simulink model "motor_controller"  (R2023b)
settings: Solver=FixedStepAuto  StartTime=0.0  StopTime=10.0  RelTol=1e-3  EnableMultiTasking=on
model workspace (MAT data in the model file):
  FOC_Ts = Simulink.Parameter
  FOC_Ts.Value = 3.65714285714e-05
  FOC_Ts.DataType = 'auto'
  FOC_Ts.Complexity = 'real'
  FOC_Ts.Dimensions = [1 1]
  Outer_Ts = Simulink.Parameter
  Outer_Ts.Value = 0.001
  Outer_Ts.DataType = 'auto'
  Outer_Ts.Complexity = 'real'
  Outer_Ts.Dimensions = [1 1]
settings Model: DataDictionary=newBoard.sldd  Creator=mfussi  LastModifiedBy=mfussi
settings SolverCC: AutoInsertRateTranBlk=on  InsertRTBMode=Never (minimum delay)
settings GRTTargetCC: CodeInterfacePackaging=Reusable function  GenerateAllocFcn=on

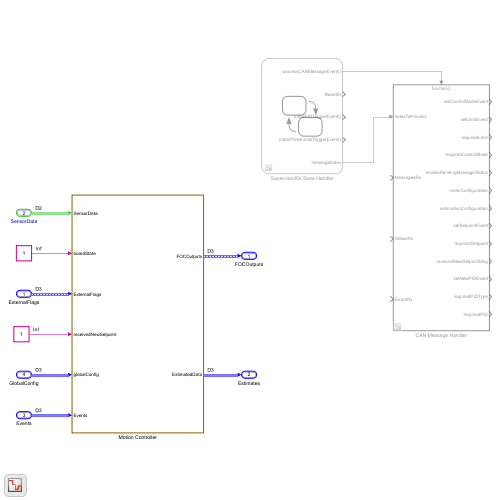
[thumbnail: Simulink's stored preview of the top-level diagram]
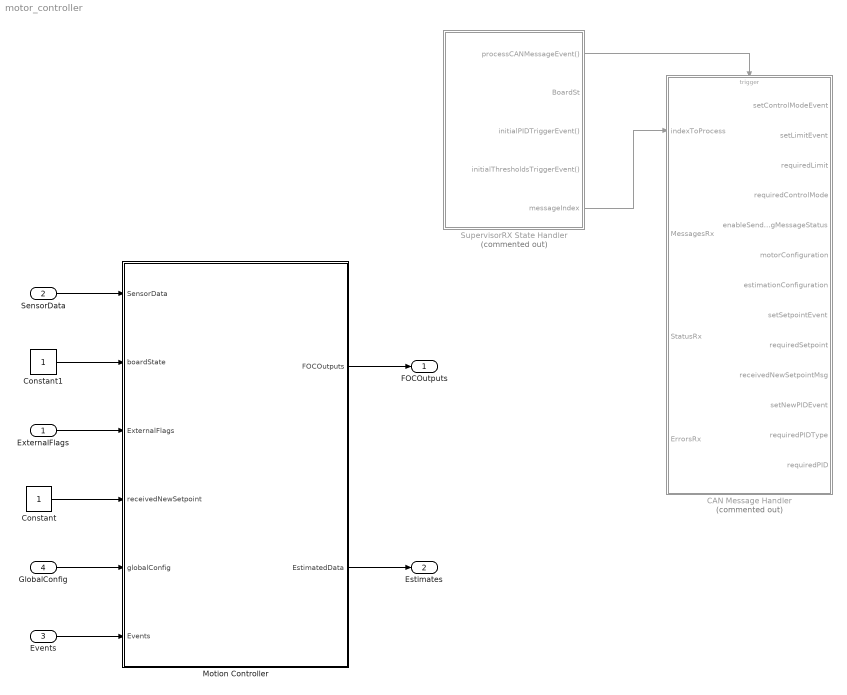
== system motor_controller ==
  ExternalFlags : Inport  OutDataTypeStr=Bus: ExternalFlags  BusOutputAsStruct=on
  SensorData : Inport  Port=2  OutDataTypeStr=Bus: SensorsData  SampleTime=FOC_Ts
  Events : Inport  Port=3  OutDataTypeStr=Bus: SupervisorReceivedEvents
  GlobalConfig : Inport  Port=4  OutDataTypeStr=Bus: GlobalConfiguration
  CAN Message Handler : Subsystem  Commented=on
  Constant : Constant  OutDataTypeStr=Inherit: Inherit via back propagation
  Constant1 : Constant
  Motion Controller : Subsystem
  SupervisorRX State Handler : Stateflow chart  Commented=on  TreatAsAtomicUnit=on
      settings: PortSchema="{\"entries\":[{\"content\":{\"sides\":[{\"content\":{},\"type\":\"ConnectorPlacement.EquallySpacedRectSide\",\"uuid\":\"4bcaed5d-410c-4a48-823b-3b1723005233\"},{\"content\":{\"connectorIds\":[\"Out3\",\"Out2\",\"Out5\",\"Out4\",\"Out1\"],\"side\":\"RIGHT\"},\"type\":\"ConnectorPlacement.EquallySpacedRectSide\",\"uuid\":\"86b3f59c-d426-4588-a6be-1a017d3ab845\"},{\"content\":{\"side\":\"TOP\"},\"type\":\"ConnectorPlacement.EquallySpacedRectSide\",\"uuid\":\"0cb05583-8f5e-45b3-ad36-5650b13dab11\"}]},\"type\":\"ConnectorPlacement.EquallySpacedConnector\",\"uuid\":\"18dc427b-0f18-405e-8b12-e70db528f537\"}],\"packageUris\":[\"http://schema.mathworks.com/mf0/Connector/R2020b\"],\"version\":\"1.0\"}"
  FOCOutputs : Outport  OutDataTypeStr=Bus: FOCOutputs
  Estimates : Outport  Port=2  OutDataTypeStr=Bus: EstimatedData
  wires:
  SupervisorRX State Handler/3(processCANMessageEvent()) -> CAN Message Handler/Trigger
  SensorData/1 -> Motion Controller/1(SensorData)
  ExternalFlags/1 -> Motion Controller/3(ExternalFlags)
  Motion Controller/1(FOCOutputs) -> FOCOutputs/1
  Motion Controller/2(EstimatedData) -> Estimates/1
  Events/1 -> Motion Controller/6(Events)
  SupervisorRX State Handler/1(messageIndex) -> CAN Message Handler/1(indexToProcess)
  GlobalConfig/1 -> Motion Controller/5(globalConfig)
  Constant/1 -> Motion Controller/4(receivedNewSetpoint)
  Constant1/1 -> Motion Controller/2(boardState)

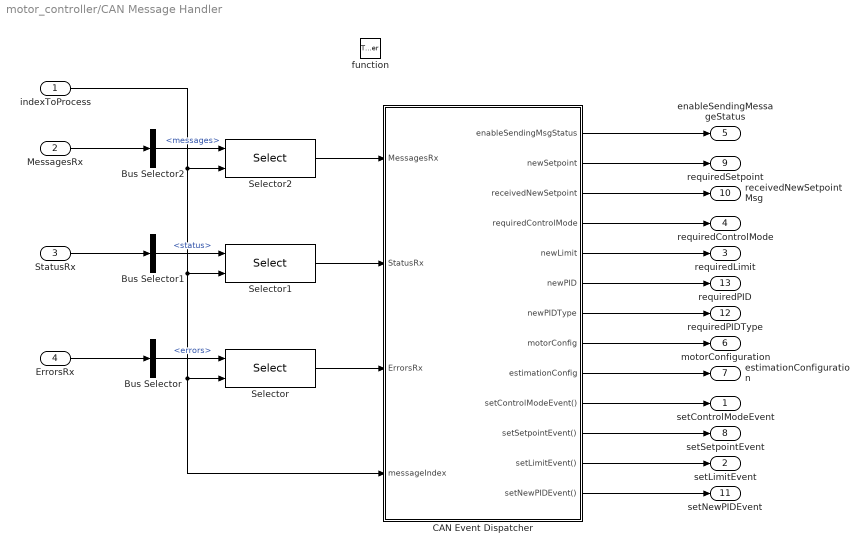
== system motor_controller/CAN Message Handler ==
  indexToProcess : Inport
  MessagesRx : Inport  Port=2  OutDataTypeStr=Bus: BUS_MESSAGES_RX_MULTIPLE
  StatusRx : Inport  Port=3  OutDataTypeStr=Bus: BUS_STATUS_RX_MULTIPLE
  ErrorsRx : Inport  Port=4  OutDataTypeStr=Bus: BUS_CAN_RX_ERRORS_MULTIPLE
  function : TriggerPort  TriggerType=function-call  VariantControl=(inherit)
  Bus Selector : BusSelector  OutputSignals=errors
  Bus Selector1 : BusSelector  OutputSignals=status
  Bus Selector2 : BusSelector  OutputSignals=messages
  CAN Event Dispatcher : Stateflow chart  TreatAsAtomicUnit=on
      settings: PortSchema="{\"entries\":[{\"content\":{\"sides\":[{\"content\":{\"connectorIds\":[\"In3\",\"In2\",\"In1\",\"In4\"]},\"type\":\"ConnectorPlacement.EquallySpacedRectSide\",\"uuid\":\"262d8322-eee9-4d2f-8394-9ad0f57315f2\"},{\"content\":{\"connectorIds\":[\"Out4\",\"Out2\",\"Out5\",\"Out1\",\"Out3\",\"Out6\",\"Out7\",\"Out8\",\"Out9\",\"Out10\",\"Out11\",\"Out12\",\"Out13\"],\"side\":\"RIGHT\"},\"type\":\"ConnectorPlacement.EquallySpacedRectSide\",\"uuid\":\"ca9d82ac-748f-4018-bf9f-4633821aba3f\"},{\"content\":{\"connectorIds\":[],\"side\":\"TOP\"},\"type\":\"ConnectorPlacement.EquallySpacedRectSide\",\"uuid\":\"6799758e-9858-4ae3-a4b1-29346dfc98be\"}]},\"type\":\"ConnectorPlacement.EquallySpacedConnector\",\"uuid\":\"ac16e6b5-85f8-470c-98ca-7de9ad02246e\"}],\"packageUris\":[\"http://schema.mathworks.com/mf0/Connector/R2020b\"],\"version\":\"1.0\"}"
  Selector : Selector  NumberOfDimensions=2  InputPortWidth=3  IndexOptions=Index vector (dialog),Index vector (port)  Indices=1,1  OutputSizes=1,1
  Selector1 : Selector  NumberOfDimensions=2  InputPortWidth=3  IndexOptions=Index vector (dialog),Index vector (port)  Indices=1,1  OutputSizes=1,1
  Selector2 : Selector  NumberOfDimensions=2  InputPortWidth=3  IndexOptions=Index vector (dialog),Index vector (port)  Indices=1,1  OutputSizes=1,1
  setControlModeEvent : Outport
  setLimitEvent : Outport  Port=2
  requiredLimit : Outport  Port=3
  requiredControlMode : Outport  Port=4
  enableSendingMessageStatus : Outport  Port=5
  motorConfiguration : Outport  Port=6  OutDataTypeStr=Bus: MotorConfig
  estimationConfiguration : Outport  Port=7  OutDataTypeStr=Bus: EstimationConfig
  setSetpointEvent : Outport  Port=8
  requiredSetpoint : Outport  Port=9
  receivedNewSetpointMsg : Outport  Port=10
  setNewPIDEvent : Outport  Port=11
  requiredPIDType : Outport  Port=12
  requiredPID : Outport  Port=13  OutDataTypeStr=Bus: BUS_MSG_PID
  wires:
  ErrorsRx/1 -> Bus Selector/1
  StatusRx/1 -> Bus Selector1/1
  MessagesRx/1 -> Bus Selector2/1
  Bus Selector2/1 -> Selector2/1  "<messages>"
  Bus Selector1/1 -> Selector1/1  "<status>"
  Bus Selector/1 -> Selector/1  "<errors>"
  indexToProcess/1 -> Selector1/2, CAN Event Dispatcher/4(messageIndex), Selector/2, Selector2/2
  Selector/1 -> CAN Event Dispatcher/1(ErrorsRx)
  Selector1/1 -> CAN Event Dispatcher/2(StatusRx)
  Selector2/1 -> CAN Event Dispatcher/3(MessagesRx)
  CAN Event Dispatcher/1(requiredControlMode) -> requiredControlMode/1
  CAN Event Dispatcher/10(setControlModeEvent()) -> setControlModeEvent/1
  CAN Event Dispatcher/11(setSetpointEvent()) -> setSetpointEvent/1
  CAN Event Dispatcher/12(setLimitEvent()) -> setLimitEvent/1
  CAN Event Dispatcher/4(enableSendingMsgStatus) -> enableSendingMessageStatus/1
  CAN Event Dispatcher/2(newSetpoint) -> requiredSetpoint/1
  CAN Event Dispatcher/3(newLimit) -> requiredLimit/1
  CAN Event Dispatcher/5(receivedNewSetpoint) -> receivedNewSetpointMsg/1
  CAN Event Dispatcher/6(newPID) -> requiredPID/1
  CAN Event Dispatcher/7(newPIDType) -> requiredPIDType/1
  CAN Event Dispatcher/8(motorConfig) -> motorConfiguration/1
  CAN Event Dispatcher/13(setNewPIDEvent()) -> setNewPIDEvent/1
  CAN Event Dispatcher/9(estimationConfig) -> estimationConfiguration/1

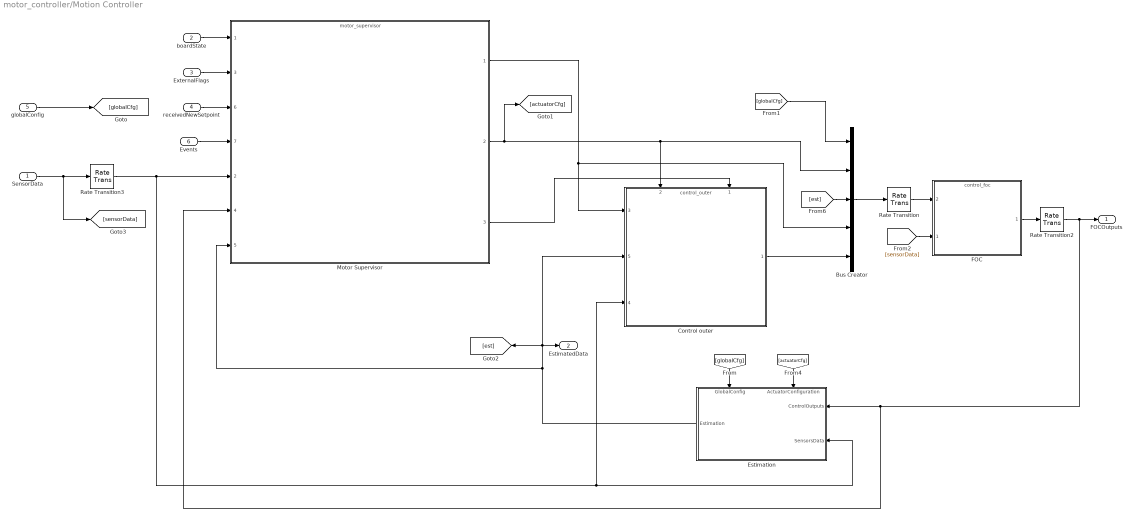
== system motor_controller/Motion Controller ==
  SensorData : Inport
  boardState : Inport  Port=2
  ExternalFlags : Inport  Port=3  OutDataTypeStr=Bus: ExternalFlags
  receivedNewSetpoint : Inport  Port=4
  globalConfig : Inport  Port=5
  Events : Inport  Port=6
  Bus Creator : BusCreator  Inputs=5  OutDataTypeStr=Bus: FOCSlowInputs  NonVirtualBus=on
      settings: InheritFromInputs=off
  Control outer : ModelReference  ModelNameDialog=control_outer.slx  SimulationMode=Normal  ModelReferenceVersion=6.7
      settings: PortSchema="{\"entries\":[{\"content\":{\"sides\":[{\"content\":{\"connectorIds\":[\"In3\",\"In5\",\"In4\"]},\"type\":\"ConnectorPlacement.EquallySpacedRectSide\",\"uuid\":\"5f0855f7-78ef-4761-b7b2-78e76d92fc4b\"},{\"content\":{\"connectorIds\":[\"Out1\"],\"side\":\"RIGHT\"},\"type\":\"ConnectorPlacement.EquallySpacedRectSide\",\"uuid\":\"ce4374cd-607c-4e0b-a8af-eb2e0e17051d\"},{\"content\":{\"connectorIds\":[\"In2\",\"In1\"],\"side\":\"TOP\"},\"type\":\"ConnectorPlacement.EquallySpacedRectSide\",\"uuid\":\"cef85d5e-e838-4f2a-8e72-80e83911c8d3\"},{\"content\":{\"side\":\"BOTTOM\"},\"type\":\"ConnectorPlacement.EquallySpacedRectSide\",\"uuid\":\"20390ec2-cce8-49cd-a78c-2a21c95dd133\"}]},\"type\":\"ConnectorPlacement.EquallySpacedConnector\",\"uuid\":\"234d6756-2ddf-48d1-9c55-249229e32550\"}],\"packageUris\":[\"http://schema.mathworks.com/mf0/Connector/R2020b\"],\"version\":\"1.0\"}"
  Estimation : Subsystem
      settings: PortSchema="{\"entries\":[{\"content\":{\"sides\":[{\"content\":{\"connectorIds\":[\"In1\",\"In2\"]},\"type\":\"ConnectorPlacement.EquallySpacedRectSide\",\"uuid\":\"180161ac-a548-41ce-8c3c-eb56a4bef2d5\"},{\"content\":{\"connectorIds\":[\"Out1\"],\"side\":\"RIGHT\"},\"type\":\"ConnectorPlacement.EquallySpacedRectSide\",\"uuid\":\"575f78f7-b1ab-47de-b691-5cd56a7f6610\"},{\"content\":{\"connectorIds\":[\"In3\",\"In4\"],\"side\":\"TOP\"},\"type\":\"ConnectorPlacement.EquallySpacedRectSide\",\"uuid\":\"318d42c0-b394-4491-8c9f-4e87fecabdd0\"}]},\"type\":\"ConnectorPlacement.EquallySpacedConnector\",\"uuid\":\"011ca5b5-9cf7-4201-870b-fa9d742ceb9c\"}],\"packageUris\":[\"http://schema.mathworks.com/mf0/Connector/R2020b\"],\"version\":\"1.0\"}"
  FOC : ModelReference  ModelNameDialog=control_foc.slx  SimulationMode=Normal  ModelReferenceVersion=6.24
      settings: PortSchema="{\"entries\":[{\"content\":{\"sides\":[{\"content\":{\"connectorIds\":[\"In2\",\"In1\"]},\"type\":\"ConnectorPlacement.EquallySpacedRectSide\",\"uuid\":\"ec9b0579-6bb0-408f-b762-24bae065c0be\"},{\"content\":{\"connectorIds\":[\"Out1\"],\"side\":\"RIGHT\"},\"type\":\"ConnectorPlacement.EquallySpacedRectSide\",\"uuid\":\"789a251a-9471-447b-a745-e431230ffa28\"},{\"content\":{\"side\":\"TOP\"},\"type\":\"ConnectorPlacement.EquallySpacedRectSide\",\"uuid\":\"ab802960-2701-40d7-b9cc-aaf192319073\"}]},\"type\":\"ConnectorPlacement.EquallySpacedConnector\",\"uuid\":\"0be03e7e-50b5-4985-b724-515ca9a23110\"}],\"packageUris\":[\"http://schema.mathworks.com/mf0/Connector/R2020b\"],\"version\":\"1.0\"}"
  Motor Supervisor : ModelReference  ModelNameDialog=motor_supervisor.slx  SimulationMode=Normal  ModelReferenceVersion=1.172
      settings: PortSchema="{\"entries\":[{\"content\":{\"sides\":[{\"content\":{\"connectorIds\":[\"In1\",\"In3\",\"In6\",\"In7\",\"In2\",\"In4\",\"In5\"]},\"type\":\"ConnectorPlacement.EquallySpacedRectSide\",\"uuid\":\"cef8e8ad-9c58-41ab-a08a-9ae722e40085\"},{\"content\":{\"connectorIds\":[\"Out1\",\"Out2\",\"Out3\"],\"side\":\"RIGHT\"},\"type\":\"ConnectorPlacement.EquallySpacedRectSide\",\"uuid\":\"f0f6bf4d-d146-4c52-85d0-e4a1fe2e14c9\"},{\"content\":{\"side\":\"TOP\"},\"type\":\"ConnectorPlacement.EquallySpacedRectSide\",\"uuid\":\"118dcde8-f32d-4dec-aaf2-5a7aa823a04d\"}]},\"type\":\"ConnectorPlacement.EquallySpacedConnector\",\"uuid\":\"5370414b-b8cf-4747-9f7c-0256206e2ab5\"}],\"packageUris\":[\"http://schema.mathworks.com/mf0/Connector/R2020b\"],\"version\":\"1.0\"}"
  Rate Transition : RateTransition  Deterministic=off  OutPortSampleTime=FOC_Ts
  Rate Transition2 : RateTransition  Deterministic=off  OutPortSampleTime=Outer_Ts
  Rate Transition3 : RateTransition  Deterministic=off  OutPortSampleTime=Outer_Ts
  FOCOutputs : Outport  OutDataTypeStr=Bus: FOCOutputs
  EstimatedData : Outport  Port=2
  wires:
  [est] -> Bus Creator/3
  Motor Supervisor/3 -> Control outer/1
  Motor Supervisor/2 -> [actuatorCfg], Bus Creator/2, Control outer/2
  Control outer/1 -> Bus Creator/5
  [actuatorCfg] -> Estimation/3(ActuatorConfiguration)
  Bus Creator/1 -> Rate Transition/1
  Estimation/1(Estimation) -> [est], Control outer/5, EstimatedData/1, Motor Supervisor/5
  Rate Transition2/1 -> Motor Supervisor/4, Estimation/1(ControlOutputs), FOCOutputs/1
  Rate Transition/1 -> FOC/2
  Motor Supervisor/1 -> Control outer/3, Bus Creator/4
  [globalCfg] -> Estimation/4(GlobalConfig)
  globalConfig/1 -> [globalCfg]
  [globalCfg] -> Bus Creator/1
  FOC/1 -> Rate Transition2/1
  Rate Transition3/1 -> Motor Supervisor/2, Control outer/4, Estimation/2(SensorsData)
  SensorData/1 -> [sensorData], Rate Transition3/1
  [sensorData] -> FOC/1
  receivedNewSetpoint/1 -> Motor Supervisor/6
  ExternalFlags/1 -> Motor Supervisor/3
  boardState/1 -> Motor Supervisor/1
  Events/1 -> Motor Supervisor/7

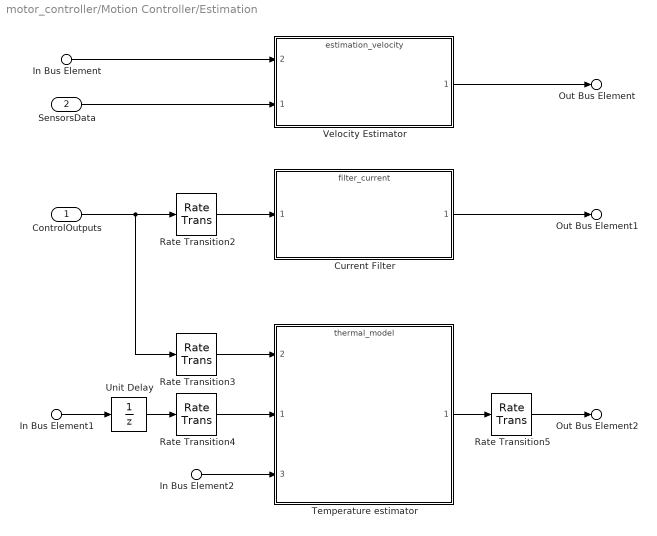
== system motor_controller/Motion Controller/Estimation ==
  ControlOutputs : Inport  OutDataTypeStr=Bus: FOCOutputs
  SensorsData : Inport  Port=2  OutDataTypeStr=Bus: SensorsData
  In Bus Element1 : Inport  Port=3  PortName=ActuatorConfiguration  Element=motor
  In Bus Element2 : Inport  Port=4  PortName=GlobalConfig  Element=estimation.environment_temperature
  In Bus Element : Inport  Port=4  PortName=GlobalConfig  Element=estimation.velocity_est_mode
  Current Filter : ModelReference  ModelNameDialog=filter_current.slx  SimulationMode=Normal  ModelReferenceVersion=6.2
  Rate Transition2 : RateTransition  Deterministic=off
  Rate Transition3 : RateTransition  Deterministic=off
  Rate Transition4 : RateTransition  Deterministic=off  OutPortSampleTime=1e-3
  Rate Transition5 : RateTransition  Deterministic=off
  Temperature estimator : ModelReference  ModelNameDialog=thermal_model.slx  SimulationMode=Normal  ModelReferenceVersion=6.10
      settings: PortSchema="{\"entries\":[{\"content\":{\"sides\":[{\"content\":{\"connectorIds\":[\"In2\",\"In1\",\"In3\"]},\"type\":\"ConnectorPlacement.EquallySpacedRectSide\",\"uuid\":\"78c786f4-5c3b-40e7-ad28-c0b961f14ec4\"},{\"content\":{\"connectorIds\":[\"Out1\"],\"side\":\"RIGHT\"},\"type\":\"ConnectorPlacement.EquallySpacedRectSide\",\"uuid\":\"b3487c62-68f2-43b6-a257-d51b1fb2e448\"},{\"content\":{\"side\":\"TOP\"},\"type\":\"ConnectorPlacement.EquallySpacedRectSide\",\"uuid\":\"5ce4df9e-b156-438c-989b-62dab6cef7f1\"}]},\"type\":\"ConnectorPlacement.EquallySpacedConnector\",\"uuid\":\"8f8c8caf-b0d2-4a2e-a596-6a6abf765763\"}],\"packageUris\":[\"http://schema.mathworks.com/mf0/Connector/R2020b\"],\"version\":\"1.0\"}"
  Unit Delay : UnitDelay  SampleTime=-1  HasFrameUpgradeWarning=on
  Velocity Estimator : ModelReference  ModelNameDialog=estimation_velocity.slx  SimulationMode=Normal  ModelReferenceVersion=6.7
      settings: PortSchema="{\"entries\":[{\"content\":{\"sides\":[{\"content\":{\"connectorIds\":[\"In2\",\"In1\"]},\"type\":\"ConnectorPlacement.EquallySpacedRectSide\",\"uuid\":\"ad3e0007-7e1a-45e3-9c4b-8557c15e59c9\"},{\"content\":{\"connectorIds\":[\"Out1\"],\"side\":\"RIGHT\"},\"type\":\"ConnectorPlacement.EquallySpacedRectSide\",\"uuid\":\"9939f2ed-714d-478a-b916-4c98246d3dad\"},{\"content\":{\"side\":\"TOP\"},\"type\":\"ConnectorPlacement.EquallySpacedRectSide\",\"uuid\":\"1f2bf02e-7550-4331-be09-78a4da3cd08c\"}]},\"type\":\"ConnectorPlacement.EquallySpacedConnector\",\"uuid\":\"c84d0359-7250-4a6f-b291-6b1b96be2690\"}],\"packageUris\":[\"http://schema.mathworks.com/mf0/Connector/R2020b\"],\"version\":\"1.0\"}"
  Out Bus Element : Outport  PortName=Estimation  Element=jointvelocities
  Out Bus Element1 : Outport  PortName=Estimation  Element=Iq_filtered
  Out Bus Element2 : Outport  PortName=Estimation  Element=motor_temperature
  wires:
  Temperature estimator/1 -> Rate Transition5/1
  Velocity Estimator/1 -> Out Bus Element/1
  Current Filter/1 -> Out Bus Element1/1
  In Bus Element1/1 -> Unit Delay/1
  SensorsData/1 -> Velocity Estimator/1
  ControlOutputs/1 -> Rate Transition2/1, Rate Transition3/1
  Rate Transition2/1 -> Current Filter/1
  Rate Transition3/1 -> Temperature estimator/2
  Rate Transition4/1 -> Temperature estimator/1
  Rate Transition5/1 -> Out Bus Element2/1
  Unit Delay/1 -> Rate Transition4/1
  In Bus Element/1 -> Velocity Estimator/2
  In Bus Element2/1 -> Temperature estimator/3

== stateflow chart motor_controller/SupervisorRX State Handler ==
  state STATE_HANDLER [parallel]
    settings: executionOrder=1
    note: ATTENTION :
        | Currently the events "BoardFaultEvent" and "OutOfBoardFaultEvent"
        | are not sent by any state. They are simple placeholder.
    state NotConfigured
      entry:
      BoardSt = BoardState.NotConfigured;
    state Fault
      entry:
      BoardSt = BoardState.Fault;
    state Configured
      entry:
      BoardSt = BoardState.Configured;
    (default) -> NotConfigured
    NotConfigured -> Fault [order 1] : BoardFaultEvent
    (junction 548) -> NotConfigured [order 1] : [!isBoardConfigured()]
    NotConfigured -> Configured [order 2] : [isBoardConfigured()]
    (junction 548) -> Configured [order 2]
    Fault -> (junction 548) : OutOfBoardFaultEvent
    Configured -> Fault : BoardFaultEvent
  state CAN_MESSAGES_FOR_LOOP [parallel]
    settings: executionOrder=2
    state state1
    (default) -> (junction 514) : {send(initialPIDTriggerEvent);
        | send(initialThresholdsTriggerEvent);}
    (junction 513) -> (junction 514)
    (junction 519) -> (junction 513)
    (junction 514) -> (junction 516) : {messageIndex = 1;}
    (junction 516) -> (junction 515) [order 1] : [messageIndex <= CAN_MAX_NUM_PACKETS]
    (junction 515) -> (junction 517) : {send(processCANMessageEvent);}
    (junction 518) -> (junction 516)
    (junction 516) -> state1 [order 2]
    (junction 517) -> (junction 518) : {messageIndex = messageIndex + 1;}
    state1 -> (junction 519)
  data: boardOk function_output boolean; messageIndex output int32; BoardSt output Enum: BoardState =BoardState.NotConfigured; CAN_MAX_NUM_PACKETS parameter
  events: BoardFaultEvent local FUNCTION_CALL_EVENT; OutOfBoardFaultEvent local FUNCTION_CALL_EVENT; processCANMessageEvent output FUNCTION_CALL_EVENT; initialThresholdsTriggerEvent output FUNCTION_CALL_EVENT; initialPIDTriggerEvent output FUNCTION_CALL_EVENT
  function boardOk=isBoardConfigured:
    | function boardOk=isBoardConfigured
    | %check here if all board services are ready 
    | boardOk=true;
    | end

== stateflow chart motor_controller/CAN Message Handler/CAN Event Dispatcher ==
  state EVENT_DISPATCHER
    state Home
    (default) -> (junction 66) : {motorConfig=InitConfParams.motorconfig;
        | estimationConfig = InitConfParams.estimationconfig;}
    (junction 87) -> (junction 66)
    (junction 66) -> (junction 69) [order 2]
    (junction 85) -> (junction 87)
    (junction 69) -> (junction 71)
    (junction 66) -> (junction 42) [order 1] : [ErrorsRx.event==false]
    (junction 42) -> (junction 111) [order 5] : [StatusRx.motor_config==true]{formatMotorConfig(); hardwareConfigMotor()}
    (junction 42) -> (junction 105) [order 4] : [StatusRx.velocity_pid==true]
        | {newPIDType = ControlModes.Velocity;
        | newPID = MessagesRx.pid;
        | send(setNewPIDEvent);}
    (junction 42) -> (junction 143) [order 6] : [StatusRx.desired_targets == true]
        | {newSetpoint = MessagesRx.desired_targets;
        | enableSendingMsgStatus = true;
        | receivedNewSetpoint = true;
        | send(setSetpointEvent);}
    (junction 42) -> (junction 50) [order 3] : [StatusRx.current_pid==true]
        | {newPIDType = ControlModes.Current;
        | newPID = MessagesRx.pid;
        | send(setNewPIDEvent);}
    (junction 42) -> (junction 48) [order 2] : [StatusRx.current_limit==true]
        | {newLimit.type = ControlModes.Current;
        | newLimit.peak = MessagesRx.current_limit.peak;
        | newLimit.nominal = MessagesRx.current_limit.nominal;
        | newLimit.overload = MessagesRx.current_limit.overload;
        | send(setLimitEvent);}
    (junction 42) -> (junction 46) [order 1] : [StatusRx.control_mode==true]
        | {requiredControlMode = convert(MessagesRx.control_mode.mode); receivedNewSetpoint=false; send(setControlModeEvent);}
    (junction 42) -> (junction 90) [order 7]
    (junction 143) -> (junction 54)
    (junction 46) -> (junction 57)
    (junction 90) -> Home
    (junction 48) -> (junction 60)
    (junction 50) -> (junction 63)
    (junction 105) -> (junction 107)
    (junction 111) -> (junction 113)
    (junction 71) -> (junction 54)
    (junction 54) -> (junction 57)
    (junction 57) -> Home
    (junction 60) -> Home
    (junction 63) -> (junction 60)
    (junction 107) -> (junction 63)
    (junction 113) -> (junction 107)
    Home -> (junction 83)
    (junction 83) -> (junction 85) [order 1] : [messageIndex == 1]{enableSendingMsgStatus = false;}
    (junction 98) -> (junction 85)
    (junction 83) -> (junction 96) [order 2]
    (junction 96) -> (junction 98)
  data: controlmode function_output Enum: ControlModes size=1; mccontrolmode function_input Enum: MCControlModes size=1; ErrorsRx input Bus: BUS_CAN_RX_ERRORS; StatusRx input Bus: BUS_STATUS_RX; MessagesRx input Bus: BUS_MESSAGES_RX; requiredControlMode output Enum: ControlModes; newSetpoint output Bus: BUS_MSG_DESIRED_TARGETS; newLimit output Bus: SV_Limits; enableSendingMsgStatus output boolean; receivedNewSetpoint output boolean =false; InitConfParams parameter Bus: ConfigurationParameters; messageIndex input int32; newPID output Bus: BUS_MSG_PID; newPIDType output Enum: ControlModes; motorConfig output Bus: MotorConfig; estimationConfig output Bus: EstimationConfig
  events: setControlModeEvent output FUNCTION_CALL_EVENT; setSetpointEvent output FUNCTION_CALL_EVENT; setLimitEvent output FUNCTION_CALL_EVENT; setNewPIDEvent output FUNCTION_CALL_EVENT
  function formatMotorConfig:
    | function formatMotorConfig
    |     %#ok<*STRNU>
    |     motorConfig.use_index = MessagesRx.motor_config.use_index;
    |     motorConfig.pole_pairs = MessagesRx.motor_config.number_poles / 2;
    |     motorConfig.encoder_tolerance = MessagesRx.motor_config.encoder_tolerance;
    |     motorConfig.rotor_encoder_resolution = MessagesRx.motor_config.rotor_encoder_resolution;
    |     motorConfig.rotor_index_offset = MessagesRx.motor_config.rotor_index_offset;
    |     motorConfig.has_quadrature_encoder = MessagesRx.motor_config.has_quadrature_encoder;
    |     motorConfig.has_hall_sens = MessagesRx.motor_config.has_hall_sens;
    |     motorConfig.has_speed_quadrature_encoder = MessagesRx.motor_config.has_speed_quadrature_encoder;
    |     motorConfig.has_torque_sens = MessagesRx.motor_config.has_torque_sens;
    |     motorConfig.enable_verbosity = MessagesRx.motor_config.enable_verbosity; 
    | end
  function hardwareConfigMotor:
    | function hardwareConfigMotor
    |     swapBC = uint8(1);
    |     hall_sens_offset = uint16(120*65536/360);
    |     
    |     rtw_configMotor(cast(motorConfig.has_quadrature_encoder, 'uint8'),...
    |                     motorConfig.rotor_encoder_resolution, ...
    |                     motorConfig.pole_pairs, ...
    |                     cast(motorConfig.has_hall_sens,'uint8'), ...
    |                     swapBC, hall_sens_offset);
    | end
  function controlmode = convert(mccontrolmode):
    | function controlmode = convert(mccontrolmode)
    | 
    |     if mccontrolmode == MCControlModes.Idle
    |         controlmode = ControlModes.Idle;
    |     elseif mccontrolmode == MCControlModes.Current
    |         controlmode = ControlModes.Current;
    |     elseif mccontrolmode == MCControlModes.SpeedVoltage
    |         controlmode = ControlModes.Velocity;
    |     elseif mccontrolmode == MCControlModes.OpenLoop
    |         controlmode = ControlModes.Voltage;
    |     else
    |         controlmode = ControlModes.Idle;
    |     end
    | 
    | end
